simulink model "zad2sim"  (R2021b)
settings: Solver=VariableStepAuto  StartTime=0.0  StopTime=10  RelTol=1e-3
values from neighbouring files (symbols this model uses):
  F = 5    [zad2dane.m]
  g = 9.81    [zad2dane.m]
  M = 0.5    [zad2dane.m]
  m = 0.2    [zad2dane.m]
undefined symbols (not defined in the file or in its folder): f, K, k
settings Model: Creator=Oskar  LastModifiedBy=Oskar

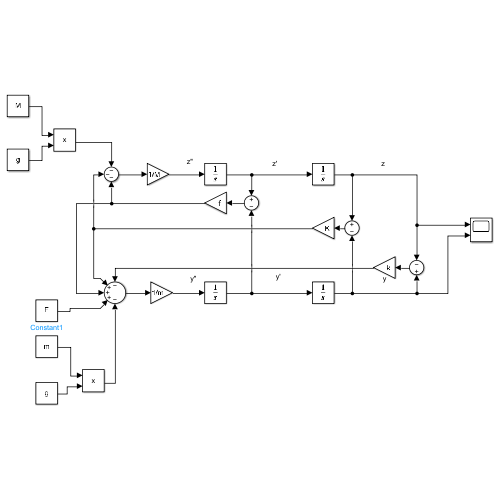
[thumbnail: Simulink's stored preview of the top-level diagram]
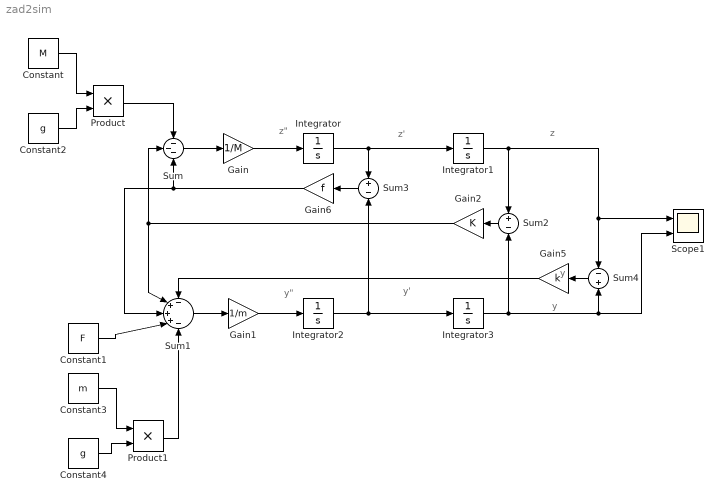
== system zad2sim ==
  note: y
  note: y'
  note: y"
  note: z
  note: z'
  note: z"
  note: y
  Constant : Constant  Value=M
  Constant1 : Constant  Value=F
  Constant2 : Constant  Value=g
  Constant3 : Constant  Value=m
  Constant4 : Constant  Value=g
  Gain : Gain  Gain=1/M
  Gain1 : Gain  Gain=1/m
  Gain2 : Gain  Gain=K
  Gain5 : Gain  Gain=k
  Gain6 : Gain  Gain=f
  Integrator : Integrator
  Integrator1 : Integrator  InitialCondition=-0.2
  Integrator2 : Integrator
  Integrator3 : Integrator  InitialCondition=-0.5
  Product : Product
  Product1 : Product
  Scope1 : Scope  NumInputPorts=2
  Sum : Sum  Inputs=---
  Sum1 : Sum  Inputs=-+++-
  Sum2 : Sum  Inputs=+|-
  Sum3 : Sum  Inputs=+|-
  Sum4 : Sum  Inputs=-|+
  wires:
  Gain1/1 -> Integrator2/1
  Sum1/1 -> Gain1/1
  Sum/1 -> Gain/1
  Gain/1 -> Integrator/1
  Integrator/1 -> Sum3/1, Integrator1/1
  Integrator1/1 -> Sum2/1, Sum4/1, Scope1/1
  Integrator2/1 -> Sum3/2, Integrator3/1
  Sum3/1 -> Gain6/1
  Sum2/1 -> Gain2/1
  Integrator3/1 -> Sum4/2, Scope1/2, Sum2/2
  Sum4/1 -> Gain5/1
  Gain6/1 -> Sum/3, Sum1/3
  Gain2/1 -> Sum/2, Sum1/2
  Constant2/1 -> Product/2
  Constant/1 -> Product/1
  Product/1 -> Sum/1
  Gain5/1 -> Sum1/1
  Constant1/1 -> Sum1/4
  Constant3/1 -> Product1/1
  Constant4/1 -> Product1/2
  Product1/1 -> Sum1/5
